simulink model "IEEE14_case"  (R2024b)
settings: Solver=FixedStepAuto  StartTime=0  StopTime=2  FixedStep=1e-7  RelTol=1e-3
values from neighbouring files (symbols this model uses):
  GFL_15_Bva = 0.009    [IEEE14_parameters.m]
  GFL_15_C_bus_pu = 7.179419    [IEEE14_parameters.m]
  GFL_15_f0 = 60    [IEEE14_parameters.m]
  GFL_15_I_id = 691.26967    [IEEE14_parameters.m]
  GFL_15_I_iq = 691.26967    [IEEE14_parameters.m]
  GFL_15_I_od = 45.2207    [IEEE14_parameters.m]
  GFL_15_I_oq = 45.2207    [IEEE14_parameters.m]
  GFL_15_I_pll = 0.78    [IEEE14_parameters.m]
  GFL_15_Kdi = 0.09    [IEEE14_parameters.m]
  GFL_15_Kdo = 0.9    [IEEE14_parameters.m]
  GFL_15_Kqi = 0.09    [IEEE14_parameters.m]
  GFL_15_Kqo = 0.9    [IEEE14_parameters.m]
  GFL_15_Lg_pu = 0.631447    [IEEE14_parameters.m]
  GFL_15_mode = 1    [IEEE14_parameters.m]
  GFL_15_P_id = 3.7166    [IEEE14_parameters.m]
  GFL_15_P_iq = 3.7166    [IEEE14_parameters.m]
  GFL_15_P_od = 0.4798    [IEEE14_parameters.m]
  GFL_15_P_oq = 0.4798    [IEEE14_parameters.m]
  GFL_15_P_pll = 290.42    [IEEE14_parameters.m]
  GFL_15_Qe_ref = 0.2    [IEEE14_parameters.m]
  GFL_15_Rg_pu = 0.024016    [IEEE14_parameters.m]
  GFL_15_Sbase = 1.000000e+4    (= 10000)    [IEEE14_parameters.m]
  GFL_15_Tdi = 0.01    [IEEE14_parameters.m]
  GFL_15_Tdo = 0.2    [IEEE14_parameters.m]
  GFL_15_Tqi = 0.01    [IEEE14_parameters.m]
  GFL_15_Tqo = 0.2    [IEEE14_parameters.m]
  GFL_15_Vbase = 380    [IEEE14_parameters.m]
  GFL_15_Vdc_ref = 1.011475    [IEEE14_parameters.m]
  GFL_15_Vdcbase = 700    [IEEE14_parameters.m]
  GFL_15_vq_ref = 0    [IEEE14_parameters.m]
  GFL_16_Bva = 0.002    [IEEE14_parameters.m]
  GFL_16_C_bus_pu = 7.179419    [IEEE14_parameters.m]
  GFL_16_f0 = 60    [IEEE14_parameters.m]
  GFL_16_I_id = 691.26967    [IEEE14_parameters.m]
  GFL_16_I_iq = 691.26967    [IEEE14_parameters.m]
  GFL_16_I_od = 45.2207    [IEEE14_parameters.m]
  GFL_16_I_oq = 45.2207    [IEEE14_parameters.m]
  GFL_16_I_pll = 0.78    [IEEE14_parameters.m]
  GFL_16_Kdi = 0.05    [IEEE14_parameters.m]
  GFL_16_Kdo = 0.5    [IEEE14_parameters.m]
  GFL_16_Kqi = 0.05    [IEEE14_parameters.m]
  GFL_16_Kqo = 0.5    [IEEE14_parameters.m]
  GFL_16_Lg_pu = 0.631447    [IEEE14_parameters.m]
  GFL_16_mode = 1    [IEEE14_parameters.m]
  GFL_16_P_id = 3.7166    [IEEE14_parameters.m]
  GFL_16_P_iq = 3.7166    [IEEE14_parameters.m]
  GFL_16_P_od = 0.4798    [IEEE14_parameters.m]
  GFL_16_P_oq = 0.4798    [IEEE14_parameters.m]
  GFL_16_P_pll = 290.42    [IEEE14_parameters.m]
  GFL_16_Qe_ref = 0.2    [IEEE14_parameters.m]
  GFL_16_Rg_pu = 0.024016    [IEEE14_parameters.m]
  GFL_16_Sbase = 1.000000e+4    (= 10000)    [IEEE14_parameters.m]
  GFL_16_Tdi = 0.01    [IEEE14_parameters.m]
  GFL_16_Tdo = 0.2    [IEEE14_parameters.m]
  GFL_16_Tqi = 0.01    [IEEE14_parameters.m]
  GFL_16_Tqo = 0.2    [IEEE14_parameters.m]
  GFL_16_Vbase = 380    [IEEE14_parameters.m]
  GFL_16_Vdc_ref = 1.01144    [IEEE14_parameters.m]
  GFL_16_Vdcbase = 700    [IEEE14_parameters.m]
  GFL_16_vq_ref = 0    [IEEE14_parameters.m]
  GFL_17_Bva = 0.002    [IEEE14_parameters.m]
  GFL_17_C_bus_pu = 7.179419    [IEEE14_parameters.m]
  GFL_17_f0 = 60    [IEEE14_parameters.m]
  GFL_17_I_id = 691.26967    [IEEE14_parameters.m]
  GFL_17_I_iq = 691.26967    [IEEE14_parameters.m]
  GFL_17_I_od = 45.2207    [IEEE14_parameters.m]
  GFL_17_I_oq = 45.2207    [IEEE14_parameters.m]
  GFL_17_I_pll = 0.78    [IEEE14_parameters.m]
  GFL_17_Kdi = 0.05    [IEEE14_parameters.m]
  GFL_17_Kdo = 0.5    [IEEE14_parameters.m]
  GFL_17_Kqi = 0.05    [IEEE14_parameters.m]
  GFL_17_Kqo = 0.5    [IEEE14_parameters.m]
  GFL_17_Lg_pu = 0.631447    [IEEE14_parameters.m]
  GFL_17_mode = 1    [IEEE14_parameters.m]
  GFL_17_P_id = 3.7166    [IEEE14_parameters.m]
  GFL_17_P_iq = 3.7166    [IEEE14_parameters.m]
  GFL_17_P_od = 0.4798    [IEEE14_parameters.m]
  GFL_17_P_oq = 0.4798    [IEEE14_parameters.m]
  GFL_17_P_pll = 290.42    [IEEE14_parameters.m]
  GFL_17_Qe_ref = 0.2    [IEEE14_parameters.m]
  GFL_17_Rg_pu = 0.024016    [IEEE14_parameters.m]
  GFL_17_Sbase = 1.000000e+4    (= 10000)    [IEEE14_parameters.m]
  GFL_17_Tdi = 0.01    [IEEE14_parameters.m]
  GFL_17_Tdo = 0.2    [IEEE14_parameters.m]
  GFL_17_Tqi = 0.01    [IEEE14_parameters.m]
  GFL_17_Tqo = 0.2    [IEEE14_parameters.m]
  GFL_17_Vbase = 380    [IEEE14_parameters.m]
  GFL_17_Vdc_ref = 1.011632    [IEEE14_parameters.m]
  GFL_17_Vdcbase = 700    [IEEE14_parameters.m]
  GFL_17_vq_ref = 0    [IEEE14_parameters.m]
  GFL_18_Bva = 0.002    [IEEE14_parameters.m]
  GFL_18_C_bus_pu = 7.179419    [IEEE14_parameters.m]
  GFL_18_f0 = 60    [IEEE14_parameters.m]
  GFL_18_I_id = 691.26967    [IEEE14_parameters.m]
  GFL_18_I_iq = 691.26967    [IEEE14_parameters.m]
  GFL_18_I_od = 45.2207    [IEEE14_parameters.m]
  GFL_18_I_oq = 45.2207    [IEEE14_parameters.m]
  GFL_18_I_pll = 0.78    [IEEE14_parameters.m]
  GFL_18_Kdi = 0.05    [IEEE14_parameters.m]
  GFL_18_Kdo = 0.5    [IEEE14_parameters.m]
  GFL_18_Kqi = 0.05    [IEEE14_parameters.m]
  GFL_18_Kqo = 0.5    [IEEE14_parameters.m]
  GFL_18_Lg_pu = 0.631447    [IEEE14_parameters.m]
  GFL_18_mode = 1    [IEEE14_parameters.m]
  GFL_18_P_id = 3.7166    [IEEE14_parameters.m]
  GFL_18_P_iq = 3.7166    [IEEE14_parameters.m]
  GFL_18_P_od = 0.4798    [IEEE14_parameters.m]
  GFL_18_P_oq = 0.4798    [IEEE14_parameters.m]
  GFL_18_P_pll = 290.42    [IEEE14_parameters.m]
  GFL_18_Qe_ref = 0.2    [IEEE14_parameters.m]
  GFL_18_Rg_pu = 0.024016    [IEEE14_parameters.m]
  GFL_18_Sbase = 1.000000e+4    (= 10000)    [IEEE14_parameters.m]
  GFL_18_Tdi = 0.01    [IEEE14_parameters.m]
  GFL_18_Tdo = 0.2    [IEEE14_parameters.m]
  GFL_18_Tqi = 0.01    [IEEE14_parameters.m]
  GFL_18_Tqo = 0.2    [IEEE14_parameters.m]
  GFL_18_Vbase = 380    [IEEE14_parameters.m]
  GFL_18_Vdc_ref = 1.011572    [IEEE14_parameters.m]
  GFL_18_Vdcbase = 700    [IEEE14_parameters.m]
  GFL_18_vq_ref = 0    [IEEE14_parameters.m]
  ... (+180 more)
(part 9 of 25)

== system IEEE14_case/AC_1/iq_bus_6_block ==
  note: iq_bus_6 in case14gfl
      | $\mathrm{iq}_{\mathrm{SG},D,6}-\mathrm{iq}_{\mathrm{load},6}+\mathrm{iq}_{\mathrm{line},5,6}-\mathrm{iq}_{\mathrm{line},6,11}-\mathrm{iq}_{\mathrm{line},6,12}-\mathrm{iq}_{\mathrm{line},6,13}$
      | Automatically generated on 2025-10-09 21:40:16 .
  Input_iq_SG_D_6_fd9b5 : Inport
  State_iq_load_6_74227 : Inport  Port=2
  State_iq_line_5_6_4236b : Inport  Port=3
  State_iq_line_6_11_dc417 : Inport  Port=4
  State_iq_line_6_12_b02a7 : Inport  Port=5
  State_iq_line_6_13_efd13 : Inport  Port=6
  Add_7536a : Sum
  Subtract_448e5 : Sum  Inputs=+-
  Subtract_74d5f : Sum  Inputs=+-
  Subtract_a35fe : Sum  Inputs=+-
  Subtract_b4e0a : Sum  Inputs=+-
  Blockout_iq_bus_6_4d630 : Outport
  wires:
  Subtract_74d5f/1 -> Subtract_b4e0a/1
  Subtract_a35fe/1 -> Subtract_74d5f/1
  Input_iq_SG_D_6_fd9b5/1 -> Subtract_448e5/1
  Subtract_448e5/1 -> Add_7536a/1
  Add_7536a/1 -> Subtract_a35fe/1
  State_iq_line_5_6_4236b/1 -> Add_7536a/2
  State_iq_load_6_74227/1 -> Subtract_448e5/2
  State_iq_line_6_11_dc417/1 -> Subtract_a35fe/2
  State_iq_line_6_12_b02a7/1 -> Subtract_74d5f/2
  State_iq_line_6_13_efd13/1 -> Subtract_b4e0a/2
  Subtract_b4e0a/1 -> Blockout_iq_bus_6_4d630/1

== system IEEE14_case/AC_1/iq_bus_7_block ==
  note: iq_bus_7 in case14gfl
      | $\mathrm{iq}_{\mathrm{line},4,7}-\mathrm{iq}_{\mathrm{line},7,8}-\mathrm{iq}_{\mathrm{line},7,9}$
      | Automatically generated on 2025-10-09 21:40:18 .
  State_iq_line_4_7_bfb83 : Inport
  State_iq_line_7_8_54428 : Inport  Port=2
  State_iq_line_7_9_fd2c4 : Inport  Port=3
  Subtract_8d108 : Sum  Inputs=+-
  Subtract_ae24a : Sum  Inputs=+-
  Blockout_iq_bus_7_85d72 : Outport
  wires:
  Subtract_8d108/1 -> Blockout_iq_bus_7_85d72/1
  State_iq_line_7_9_fd2c4/1 -> Subtract_8d108/2
  State_iq_line_4_7_bfb83/1 -> Subtract_ae24a/1
  State_iq_line_7_8_54428/1 -> Subtract_ae24a/2
  Subtract_ae24a/1 -> Subtract_8d108/1

== system IEEE14_case/AC_1/iq_bus_8_block ==
  note: iq_bus_8 in case14gfl
      | $\mathrm{iq}_{\mathrm{SG},D,8}+\mathrm{iq}_{\mathrm{line},7,8}$
      | Automatically generated on 2025-10-09 21:40:20 .
  Input_iq_SG_D_8_05cc5 : Inport
  State_iq_line_7_8_02a2e : Inport  Port=2
  Add_2cb00 : Sum
  Blockout_iq_bus_8_a9e89 : Outport
  wires:
  Add_2cb00/1 -> Blockout_iq_bus_8_a9e89/1
  State_iq_line_7_8_02a2e/1 -> Add_2cb00/2
  Input_iq_SG_D_8_05cc5/1 -> Add_2cb00/1

== system IEEE14_case/AC_1/iq_bus_9_block ==
  note: iq_bus_9 in case14gfl
      | $\mathrm{iq}_{\mathrm{line},4,9}-\mathrm{iq}_{\mathrm{load},9}+\mathrm{iq}_{\mathrm{line},7,9}-\mathrm{iq}_{\mathrm{line},9,10}-\mathrm{iq}_{\mathrm{line},9,14}$
      | Automatically generated on 2025-10-09 21:40:22 .
  State_iq_load_9_b0a53 : Inport
  State_iq_line_4_9_4d417 : Inport  Port=2
  State_iq_line_7_9_360e6 : Inport  Port=3
  State_iq_line_9_10_294ee : Inport  Port=4
  State_iq_line_9_14_10f53 : Inport  Port=5
  Add_23a6a : Sum
  Add_e8f35 : Sum
  Constant_-1_d914d : Constant  Value=-1
  Product_e44f7 : Product
  Subtract_3c9e7 : Sum  Inputs=+-
  Subtract_96d13 : Sum  Inputs=+-
  Blockout_iq_bus_9_d3dd5 : Outport
  wires:
  Constant_-1_d914d/1 -> Product_e44f7/1
  Product_e44f7/1 -> Add_23a6a/1
  Add_23a6a/1 -> Add_e8f35/1
  State_iq_line_4_9_4d417/1 -> Add_23a6a/2
  State_iq_load_9_b0a53/1 -> Product_e44f7/2
  State_iq_line_7_9_360e6/1 -> Add_e8f35/2
  Add_e8f35/1 -> Subtract_96d13/1
  State_iq_line_9_10_294ee/1 -> Subtract_96d13/2
  Subtract_96d13/1 -> Subtract_3c9e7/1
  State_iq_line_9_14_10f53/1 -> Subtract_3c9e7/2
  Subtract_3c9e7/1 -> Blockout_iq_bus_9_d3dd5/1

== system IEEE14_case/AC_1/vd_bus_15_out_block ==
  note: vd_bus_15_out in case14gfl
      | $\mathrm{vd}_{\mathrm{bus},15}$
      | Automatically generated on 2025-10-09 21:40:32 .
  State_vd_bus_15_8a646 : Inport
  Blockout_vd_bus_15_out_53236 : Outport
  wires:
  State_vd_bus_15_8a646/1 -> Blockout_vd_bus_15_out_53236/1

== system IEEE14_case/AC_1/vd_bus_16_out_block ==
  note: vd_bus_16_out in case14gfl
      | $\mathrm{vd}_{\mathrm{bus},16}$
      | Automatically generated on 2025-10-09 21:40:34 .
  State_vd_bus_16_c68f5 : Inport
  Blockout_vd_bus_16_out_bf920 : Outport
  wires:
  State_vd_bus_16_c68f5/1 -> Blockout_vd_bus_16_out_bf920/1

== system IEEE14_case/AC_1/vd_bus_17_out_block ==
  note: vd_bus_17_out in case14gfl
      | $\mathrm{vd}_{\mathrm{bus},17}$
      | Automatically generated on 2025-10-09 21:40:37 .
  State_vd_bus_17_d959d : Inport
  Blockout_vd_bus_17_out_ee528 : Outport
  wires:
  State_vd_bus_17_d959d/1 -> Blockout_vd_bus_17_out_ee528/1

== system IEEE14_case/AC_1/vd_bus_18_out_block ==
  note: vd_bus_18_out in case14gfl
      | $\mathrm{vd}_{\mathrm{bus},18}$
      | Automatically generated on 2025-10-09 21:40:40 .
  State_vd_bus_18_46c9f : Inport
  Blockout_vd_bus_18_out_c2e2f : Outport
  wires:
  State_vd_bus_18_46c9f/1 -> Blockout_vd_bus_18_out_c2e2f/1

== system IEEE14_case/AC_1/vd_bus_1_out_block ==
  note: vd_bus_1_out in case14gfl
      | $\mathrm{vd}_{\mathrm{bus},1}$
      | Automatically generated on 2025-10-09 21:40:02 .
  State_vd_bus_1_5dc0e : Inport
  Blockout_vd_bus_1_out_41eef : Outport
  wires:
  State_vd_bus_1_5dc0e/1 -> Blockout_vd_bus_1_out_41eef/1

== system IEEE14_case/AC_1/vd_bus_2_out_block ==
  note: vd_bus_2_out in case14gfl
      | $\mathrm{vd}_{\mathrm{bus},2}$
      | Automatically generated on 2025-10-09 21:40:04 .
  State_vd_bus_2_3f94d : Inport
  Blockout_vd_bus_2_out_d1efc : Outport
  wires:
  State_vd_bus_2_3f94d/1 -> Blockout_vd_bus_2_out_d1efc/1

== system IEEE14_case/AC_1/vd_bus_3_out_block ==
  note: vd_bus_3_out in case14gfl
      | $\mathrm{vd}_{\mathrm{bus},3}$
      | Automatically generated on 2025-10-09 21:40:07 .
  State_vd_bus_3_4d21d : Inport
  Blockout_vd_bus_3_out_e3de8 : Outport
  wires:
  State_vd_bus_3_4d21d/1 -> Blockout_vd_bus_3_out_e3de8/1

== system IEEE14_case/AC_1/vd_bus_6_out_block ==
  note: vd_bus_6_out in case14gfl
      | $\mathrm{vd}_{\mathrm{bus},6}$
      | Automatically generated on 2025-10-09 21:40:14 .
  State_vd_bus_6_a4f60 : Inport
  Blockout_vd_bus_6_out_fb39e : Outport
  wires:
  State_vd_bus_6_a4f60/1 -> Blockout_vd_bus_6_out_fb39e/1

== system IEEE14_case/AC_1/vd_bus_8_out_block ==
  note: vd_bus_8_out in case14gfl
      | $\mathrm{vd}_{\mathrm{bus},8}$
      | Automatically generated on 2025-10-09 21:40:18 .
  State_vd_bus_8_bc007 : Inport
  Blockout_vd_bus_8_out_d3476 : Outport
  wires:
  State_vd_bus_8_bc007/1 -> Blockout_vd_bus_8_out_d3476/1

== system IEEE14_case/AC_1/vq_bus_15_out_block ==
  note: vq_bus_15_out in case14gfl
      | $\mathrm{vq}_{\mathrm{bus},15}$
      | Automatically generated on 2025-10-09 21:40:32 .
  State_vq_bus_15_e85b0 : Inport
  Blockout_vq_bus_15_out_b5487 : Outport
  wires:
  State_vq_bus_15_e85b0/1 -> Blockout_vq_bus_15_out_b5487/1

== system IEEE14_case/AC_1/vq_bus_16_out_block ==
  note: vq_bus_16_out in case14gfl
      | $\mathrm{vq}_{\mathrm{bus},16}$
      | Automatically generated on 2025-10-09 21:40:35 .
  State_vq_bus_16_bbd15 : Inport
  Blockout_vq_bus_16_out_7f446 : Outport
  wires:
  State_vq_bus_16_bbd15/1 -> Blockout_vq_bus_16_out_7f446/1

== system IEEE14_case/AC_1/vq_bus_17_out_block ==
  note: vq_bus_17_out in case14gfl
      | $\mathrm{vq}_{\mathrm{bus},17}$
      | Automatically generated on 2025-10-09 21:40:37 .
  State_vq_bus_17_ceb31 : Inport
  Blockout_vq_bus_17_out_c5b42 : Outport
  wires:
  State_vq_bus_17_ceb31/1 -> Blockout_vq_bus_17_out_c5b42/1

== system IEEE14_case/AC_1/vq_bus_18_out_block ==
  note: vq_bus_18_out in case14gfl
      | $\mathrm{vq}_{\mathrm{bus},18}$
      | Automatically generated on 2025-10-09 21:40:40 .
  State_vq_bus_18_e31db : Inport
  Blockout_vq_bus_18_out_45376 : Outport
  wires:
  State_vq_bus_18_e31db/1 -> Blockout_vq_bus_18_out_45376/1

== system IEEE14_case/AC_1/vq_bus_1_out_block ==
  note: vq_bus_1_out in case14gfl
      | $\mathrm{vq}_{\mathrm{bus},1}$
      | Automatically generated on 2025-10-09 21:40:03 .
  State_vq_bus_1_00178 : Inport
  Blockout_vq_bus_1_out_08423 : Outport
  wires:
  State_vq_bus_1_00178/1 -> Blockout_vq_bus_1_out_08423/1

== system IEEE14_case/AC_1/vq_bus_2_out_block ==
  note: vq_bus_2_out in case14gfl
      | $\mathrm{vq}_{\mathrm{bus},2}$
      | Automatically generated on 2025-10-09 21:40:05 .
  State_vq_bus_2_ea0d1 : Inport
  Blockout_vq_bus_2_out_c2eb9 : Outport
  wires:
  State_vq_bus_2_ea0d1/1 -> Blockout_vq_bus_2_out_c2eb9/1

== system IEEE14_case/AC_1/vq_bus_3_out_block ==
  note: vq_bus_3_out in case14gfl
      | $\mathrm{vq}_{\mathrm{bus},3}$
      | Automatically generated on 2025-10-09 21:40:08 .
  State_vq_bus_3_c1e3e : Inport
  Blockout_vq_bus_3_out_bf333 : Outport
  wires:
  State_vq_bus_3_c1e3e/1 -> Blockout_vq_bus_3_out_bf333/1

== system IEEE14_case/AC_1/vq_bus_6_out_block ==
  note: vq_bus_6_out in case14gfl
      | $\mathrm{vq}_{\mathrm{bus},6}$
      | Automatically generated on 2025-10-09 21:40:14 .
  State_vq_bus_6_b99ed : Inport
  Blockout_vq_bus_6_out_b9abb : Outport
  wires:
  State_vq_bus_6_b99ed/1 -> Blockout_vq_bus_6_out_b9abb/1

== system IEEE14_case/AC_1/vq_bus_8_out_block ==
  note: vq_bus_8_out in case14gfl
      | $\mathrm{vq}_{\mathrm{bus},8}$
      | Automatically generated on 2025-10-09 21:40:19 .
  State_vq_bus_8_b3a86 : Inport
  Blockout_vq_bus_8_out_36371 : Outport
  wires:
  State_vq_bus_8_b3a86/1 -> Blockout_vq_bus_8_out_36371/1

== system IEEE14_case/GFL_15/d_Idv_GFL_15_block ==
  note: d_Idv_GFL_15 in case14gfl
      | $-\frac{\mathrm{Idv}_{\mathrm{GFL},15}+\mathrm{Kdo}\,\left(\mathrm{Vbase}\,\left(v_{q,\mathrm{GFL},15}\,\cos\left(\theta _{\mathrm{pll},\mathrm{GFL},15}\right)+v_{d,\mathrm{GFL},15}\,\sin\left(\theta _{\mathrm{pll},\mathrm{GFL},15}\right)\right)+\frac{\Psi _{d,\mathrm{GFL},15}+\mathrm{Kdi}\,\mathrm{Vbase}\,\left(v_{q,\mathrm{GFL},15}\,\cos\left(\theta _{\mathrm{pll},\mathrm{GFL},15}\right)+v_{d,\mathrm{GFL},15}\,\sin\left(\theta _{\mathrm{pll},\mathrm{GFL},15}\right)\right)}{\mathrm{Tdi}}\right)}{\mathrm{Tdo}}$
      | Automatically generated on 2025-10-09 21:35:26 .
  State_Idv_GFL_15_ca6d1 : Inport
  Input_v_d_GFL_15_d6ef0 : Inport  Port=2
  State_theta_pll_GFL_15_12ffd : Inport  Port=3
  Input_v_q_GFL_15_617c4 : Inport  Port=4
  State_theta_pll_GFL_15_9725f : Inport  Port=5
  Input_v_d_GFL_15_adaa4 : Inport  Port=6
  State_theta_pll_GFL_15_963fe : Inport  Port=7
  Input_v_q_GFL_15_86e6c : Inport  Port=8
  State_theta_pll_GFL_15_2202b : Inport  Port=9
  State_Psi_d_GFL_15_22a12 : Inport  Port=10
  Add_30c23 : Sum
  Add_6e6b0 : Sum
  Add_ecf0e : Sum
  Add_ed6d2 : Sum
  Constant_-1_8c527 : Constant  Value=-1
  Constant_-1_bad54 : Constant  Value=-1
  Constant_-1_d2cc2 : Constant  Value=-1
  Constant_Kdi_3c48e : Constant  Value=Kdi
  Constant_Kdo_c5a85 : Constant  Value=Kdo
  Constant_Tdi_93e84 : Constant  Value=Tdi
  Constant_Tdo_322af : Constant  Value=Tdo
  Constant_Vbase_69f49 : Constant  Value=Vbase
  Constant_Vbase_8e2e0 : Constant  Value=Vbase
  Divide_08330 : Product  Inputs=*/
  Divide_106bd : Product  Inputs=*/
  MathFunc_cos_6a27c : Trigonometry  Operator=cos
  MathFunc_cos_b8fe7 : Trigonometry  Operator=cos
  MathFunc_sin_2b1dd : Trigonometry
  MathFunc_sin_32677 : Trigonometry
  Product_134c0 : Product
  Product_1d184 : Product
  Product_32e14 : Product
  Product_6e7d5 : Product
  Product_75262 : Product
  Product_a160a : Product
  Product_ae5a0 : Product
  Product_beb8a : Product
  Product_d484f : Product
  Product_e74b0 : Product
  Product_f9eeb : Product
  Subtract_37e01 : Sum  Inputs=+-
  Blockout_d_Idv_GFL_15_06d8e : Outport
  wires:
  Add_30c23/1 -> Divide_106bd/1
  State_theta_pll_GFL_15_963fe/1 -> MathFunc_sin_2b1dd/1
  MathFunc_sin_2b1dd/1 -> Product_ae5a0/2
  State_theta_pll_GFL_15_2202b/1 -> MathFunc_cos_6a27c/1
  MathFunc_cos_6a27c/1 -> Product_a160a/2
  Product_1d184/1 -> Add_ed6d2/1
  Constant_Kdi_3c48e/1 -> Product_134c0/2
  Constant_-1_bad54/1 -> Product_134c0/1
  Product_ae5a0/1 -> Add_ecf0e/1
  Input_v_d_GFL_15_adaa4/1 -> Product_ae5a0/1
  Input_v_q_GFL_15_86e6c/1 -> Product_a160a/1
  MathFunc_sin_32677/1 -> Product_1d184/2
  State_theta_pll_GFL_15_12ffd/1 -> MathFunc_sin_32677/1
  State_theta_pll_GFL_15_9725f/1 -> MathFunc_cos_b8fe7/1
  State_Idv_GFL_15_ca6d1/1 -> Product_e74b0/2
  Product_134c0/1 -> Product_32e14/1
  Input_v_d_GFL_15_d6ef0/1 -> Product_1d184/1
  Constant_Vbase_8e2e0/1 -> Product_32e14/2
  Product_a160a/1 -> Add_ecf0e/2
  Input_v_q_GFL_15_617c4/1 -> Product_beb8a/1
  MathFunc_cos_b8fe7/1 -> Product_beb8a/2
  Product_32e14/1 -> Product_d484f/1
  Add_ecf0e/1 -> Product_d484f/2
  Constant_-1_d2cc2/1 -> Product_f9eeb/1
  Constant_Vbase_69f49/1 -> Product_f9eeb/2
  Product_beb8a/1 -> Add_ed6d2/2
  Product_d484f/1 -> Subtract_37e01/1
  State_Psi_d_GFL_15_22a12/1 -> Subtract_37e01/2
  Product_f9eeb/1 -> Product_6e7d5/1
  Add_ed6d2/1 -> Product_6e7d5/2
  Subtract_37e01/1 -> Divide_08330/1
  Constant_Tdi_93e84/1 -> Divide_08330/2
  Product_6e7d5/1 -> Add_6e6b0/1
  Divide_08330/1 -> Add_6e6b0/2
  Constant_-1_8c527/1 -> Product_e74b0/1
  Product_75262/1 -> Add_30c23/2
  Constant_Kdo_c5a85/1 -> Product_75262/1
  Add_6e6b0/1 -> Product_75262/2
  Product_e74b0/1 -> Add_30c23/1
  Constant_Tdo_322af/1 -> Divide_106bd/2
  Divide_106bd/1 -> Blockout_d_Idv_GFL_15_06d8e/1

== system IEEE14_case/GFL_15/d_Iqv_GFL_15_block ==
  note: d_Iqv_GFL_15 in case14gfl
      | $-\frac{\mathrm{Iqv}_{\mathrm{GFL},15}-\mathrm{Kqo}\,\left(\mathrm{Vbase}\,\left(v_{d,\mathrm{GFL},15}\,\cos\left(\theta _{\mathrm{pll},\mathrm{GFL},15}\right)-v_{q,\mathrm{GFL},15}\,\sin\left(\theta _{\mathrm{pll},\mathrm{GFL},15}\right)\right)-\frac{\Psi _{q,\mathrm{GFL},15}-\mathrm{Kqi}\,\mathrm{Vbase}\,\left(v_{d,\mathrm{GFL},15}\,\cos\left(\theta _{\mathrm{pll},\mathrm{GFL},15}\right)-v_{q,\mathrm{GFL},15}\,\sin\left(\theta _{\mathrm{pll},\mathrm{GFL},15}\right)\right)}{\mathrm{Tqi}}\right)}{\mathrm{Tqo}}$
      | Automatically generated on 2025-10-09 21:35:28 .
  State_Iqv_GFL_15_a0efa : Inport
  Input_v_d_GFL_15_e9447 : Inport  Port=2
  State_theta_pll_GFL_15_5bce6 : Inport  Port=3
  Input_v_q_GFL_15_4a34b : Inport  Port=4
  State_theta_pll_GFL_15_c6881 : Inport  Port=5
  Input_v_d_GFL_15_7c93a : Inport  Port=6
  State_theta_pll_GFL_15_e8e0d : Inport  Port=7
  Input_v_q_GFL_15_924af : Inport  Port=8
  State_theta_pll_GFL_15_f624d : Inport  Port=9
  State_Psi_q_GFL_15_d75c1 : Inport  Port=10
  Add_7b66c : Sum
  Add_cf612 : Sum
  Constant_-1_c7459 : Constant  Value=-1
  Constant_Kqi_42f9e : Constant  Value=Kqi
  Constant_Kqo_97ec0 : Constant  Value=Kqo
  Constant_Tqi_2e3dc : Constant  Value=Tqi
  Constant_Tqo_731e7 : Constant  Value=Tqo
  Constant_Vbase_41c60 : Constant  Value=Vbase
  Constant_Vbase_700be : Constant  Value=Vbase
  Divide_61f05 : Product  Inputs=*/
  Divide_b950e : Product  Inputs=*/
  MathFunc_cos_3c92d : Trigonometry  Operator=cos
  MathFunc_cos_c5429 : Trigonometry  Operator=cos
  MathFunc_sin_3ae11 : Trigonometry
  MathFunc_sin_e36a9 : Trigonometry
  Product_13c48 : Product
  Product_2727d : Product
  Product_2c1de : Product
  Product_3cbec : Product
  Product_5de87 : Product
  Product_6c92d : Product
  Product_9c883 : Product
  Product_b238b : Product
  Product_e1ab8 : Product
  Subtract_15861 : Sum  Inputs=+-
  Subtract_84f7c : Sum  Inputs=+-
  Subtract_94af4 : Sum  Inputs=+-
  Blockout_d_Iqv_GFL_15_65918 : Outport
  wires:
  MathFunc_cos_c5429/1 -> Product_5de87/2
  State_theta_pll_GFL_15_5bce6/1 -> MathFunc_cos_c5429/1
  State_theta_pll_GFL_15_e8e0d/1 -> MathFunc_cos_3c92d/1
  MathFunc_sin_3ae11/1 -> Product_b238b/2
  State_theta_pll_GFL_15_c6881/1 -> MathFunc_sin_3ae11/1
  Product_13c48/1 -> Add_7b66c/2
  State_theta_pll_GFL_15_f624d/1 -> MathFunc_sin_e36a9/1
  MathFunc_sin_e36a9/1 -> Product_3cbec/2
  Product_6c92d/1 -> Subtract_15861/1
  Input_v_d_GFL_15_7c93a/1 -> Product_6c92d/1
  MathFunc_cos_3c92d/1 -> Product_6c92d/2
  Product_3cbec/1 -> Subtract_15861/2
  Input_v_q_GFL_15_924af/1 -> Product_3cbec/1
  Product_2727d/1 -> Product_e1ab8/1
  Constant_Kqi_42f9e/1 -> Product_2727d/1
  Constant_Vbase_700be/1 -> Product_2727d/2
  Product_5de87/1 -> Subtract_84f7c/1
  Input_v_d_GFL_15_e9447/1 -> Product_5de87/1
  Input_v_q_GFL_15_4a34b/1 -> Product_b238b/1
  Subtract_15861/1 -> Product_e1ab8/2
  Product_b238b/1 -> Subtract_84f7c/2
  Product_e1ab8/1 -> Subtract_94af4/1
  State_Psi_q_GFL_15_d75c1/1 -> Subtract_94af4/2
  Constant_Vbase_41c60/1 -> Product_9c883/1
  Subtract_84f7c/1 -> Product_9c883/2
  Subtract_94af4/1 -> Divide_b950e/1
  Constant_Tqi_2e3dc/1 -> Divide_b950e/2
  Product_9c883/1 -> Add_cf612/1
  Divide_b950e/1 -> Add_cf612/2
  Constant_-1_c7459/1 -> Product_2c1de/1
  State_Iqv_GFL_15_a0efa/1 -> Product_2c1de/2
  Constant_Kqo_97ec0/1 -> Product_13c48/1
  Add_cf612/1 -> Product_13c48/2
  Divide_61f05/1 -> Blockout_d_Iqv_GFL_15_65918/1
  Product_2c1de/1 -> Add_7b66c/1
  Add_7b66c/1 -> Divide_61f05/1
  Constant_Tqo_731e7/1 -> Divide_61f05/2

== system IEEE14_case/GFL_15/d_Phi_ga_GFL_15_block ==
  note: d_Phi_ga_GFL_15 in case14gfl
      | $I_{\mathrm{od}}\,\left(V_{\mathrm{dc},\mathrm{GFL},15}-\mathrm{Vdcbase}\,\mathrm{Vdc}_{\mathrm{ref}}\right)$
      | Automatically generated on 2025-10-09 21:35:14 .
  State_V_dc_GFL_15_371a8 : Inport
  Constant_I_od_53ece : Constant  Value=I_od
  Constant_Vdc_ref_e5ef2 : Constant  Value=Vdc_ref
  Constant_Vdcbase_c0f83 : Constant  Value=Vdcbase
  Product_b2d23 : Product
  Product_c5cd1 : Product
  Subtract_28544 : Sum  Inputs=+-
  Blockout_d_Phi_ga_GFL_15_ed294 : Outport
  wires:
  Product_c5cd1/1 -> Blockout_d_Phi_ga_GFL_15_ed294/1
  Product_b2d23/1 -> Subtract_28544/2
  Constant_Vdc_ref_e5ef2/1 -> Product_b2d23/1
  Constant_Vdcbase_c0f83/1 -> Product_b2d23/2
  Constant_I_od_53ece/1 -> Product_c5cd1/1
  State_V_dc_GFL_15_371a8/1 -> Subtract_28544/1
  Subtract_28544/1 -> Product_c5cd1/2

== system IEEE14_case/GFL_15/d_Phi_gb_GFL_15_block ==
  note: d_Phi_gb_GFL_15 in case14gfl
      | $I_{\mathrm{id}}\,\left(\mathrm{Idv}_{\mathrm{GFL},15}+\Phi _{\mathrm{ga},\mathrm{GFL},15}-i_{\mathrm{gd},\mathrm{GFL},15}+P_{\mathrm{od}}\,\left(V_{\mathrm{dc},\mathrm{GFL},15}-\mathrm{Vdcbase}\,\mathrm{Vdc}_{\mathrm{ref}}\right)-\mathrm{Bva}\,\mathrm{Vbase}\,\left(v_{d,\mathrm{GFL},15}\,\cos\left(\theta _{\mathrm{pll},\mathrm{GFL},15}\right)-v_{q,\mathrm{GFL},15}\,\sin\left(\theta _{\mathrm{pll},\mathrm{GFL},15}\right)\right)\right)$
      | Automatically generated on 2025-10-09 21:35:15 .
  Input_v_d_GFL_15_ba16a : Inport
  State_theta_pll_GFL_15_82324 : Inport  Port=2
  Input_v_q_GFL_15_e2248 : Inport  Port=3
  State_theta_pll_GFL_15_58522 : Inport  Port=4
  State_Idv_GFL_15_4c70c : Inport  Port=5
  State_V_dc_GFL_15_cf545 : Inport  Port=6
  State_Phi_ga_GFL_15_778c9 : Inport  Port=7
  State_i_gd_GFL_15_ca8ed : Inport  Port=8
  Add_7f088 : Sum
  Add_ba3ac : Sum
  Add_cab57 : Sum
  Constant_-1_d2a66 : Constant  Value=-1
  Constant_Bva_25216 : Constant  Value=Bva
  Constant_I_id_90b40 : Constant  Value=I_id
  Constant_P_od_b2591 : Constant  Value=P_od
  Constant_Vbase_4f081 : Constant  Value=Vbase
  Constant_Vdc_ref_8d8d4 : Constant  Value=Vdc_ref
  Constant_Vdcbase_e266d : Constant  Value=Vdcbase
  MathFunc_cos_073c5 : Trigonometry  Operator=cos
  MathFunc_sin_6f8a0 : Trigonometry
  Product_24fb4 : Product
  Product_2f798 : Product
  Product_574fd : Product
  Product_5845e : Product
  Product_75092 : Product
  Product_77499 : Product
  Product_b1701 : Product
  Product_c7754 : Product
  Subtract_311fa : Sum  Inputs=+-
  Subtract_429b0 : Sum  Inputs=+-
  Subtract_9a423 : Sum  Inputs=+-
  Blockout_d_Phi_gb_GFL_15_f24ee : Outport
  wires:
  MathFunc_cos_073c5/1 -> Product_c7754/2
  State_theta_pll_GFL_15_82324/1 -> MathFunc_cos_073c5/1
  State_theta_pll_GFL_15_58522/1 -> MathFunc_sin_6f8a0/1
  MathFunc_sin_6f8a0/1 -> Product_24fb4/2
  Product_24fb4/1 -> Subtract_9a423/2
  Input_v_q_GFL_15_e2248/1 -> Product_24fb4/1
  Product_5845e/1 -> Product_75092/1
  Constant_-1_d2a66/1 -> Product_5845e/1
  Constant_Bva_25216/1 -> Product_5845e/2
  State_Phi_ga_GFL_15_778c9/1 -> Add_ba3ac/2
  Product_c7754/1 -> Subtract_9a423/1
  Input_v_d_GFL_15_ba16a/1 -> Product_c7754/1
  Constant_Vbase_4f081/1 -> Product_75092/2
  Product_b1701/1 -> Subtract_429b0/2
  Constant_Vdc_ref_8d8d4/1 -> Product_b1701/1
  Constant_Vdcbase_e266d/1 -> Product_b1701/2
  Product_75092/1 -> Product_77499/1
  Subtract_9a423/1 -> Product_77499/2
  Subtract_429b0/1 -> Product_2f798/2
  State_V_dc_GFL_15_cf545/1 -> Subtract_429b0/1
  Product_77499/1 -> Add_cab57/1
  State_Idv_GFL_15_4c70c/1 -> Add_cab57/2
  Product_2f798/1 -> Add_7f088/2
  Constant_P_od_b2591/1 -> Product_2f798/1
  Add_cab57/1 -> Add_7f088/1
  Add_7f088/1 -> Add_ba3ac/1
  Add_ba3ac/1 -> Subtract_311fa/1
  State_i_gd_GFL_15_ca8ed/1 -> Subtract_311fa/2
  Constant_I_id_90b40/1 -> Product_574fd/1
  Subtract_311fa/1 -> Product_574fd/2
  Product_574fd/1 -> Blockout_d_Phi_gb_GFL_15_f24ee/1

== system IEEE14_case/GFL_15/d_Phi_gc_GFL_15_block ==
  note: d_Phi_gc_GFL_15 in case14gfl
      | $-I_{\mathrm{oq}}\,\left(\mathrm{Qe}_{\mathrm{ref}}\,\mathrm{Sbase}+1.73205080756888\,\mathrm{Vbase}\,i_{\mathrm{gd},\mathrm{GFL},15}\,\left(v_{q,\mathrm{GFL},15}\,\cos\left(\theta _{\mathrm{pll},\mathrm{GFL},15}\right)+v_{d,\mathrm{GFL},15}\,\sin\left(\theta _{\mathrm{pll},\mathrm{GFL},15}\right)\right)+1.73205080756888\,\mathrm{Vbase}\,i_{\mathrm{gq},\mathrm{GFL},15}\,\left(v_{d,\mathrm{GFL},15}\,\cos\left(\theta _{\mathrm{pll},\mathrm{GFL},15}\right)-v_{q,\mathrm{GFL},15}\,\sin\left(\theta _{\mathrm{pll},\mathrm{GFL},15}\right)\right)\right)$
      | Automatically generated on 2025-10-09 21:35:18 .
  State_i_gd_GFL_15_68d30 : Inport
  Input_v_d_GFL_15_05f07 : Inport  Port=2
  State_theta_pll_GFL_15_5b93f : Inport  Port=3
  Input_v_q_GFL_15_7ae45 : Inport  Port=4
  State_theta_pll_GFL_15_647bc : Inport  Port=5
  State_i_gq_GFL_15_2aff2 : Inport  Port=6
  Input_v_d_GFL_15_b97ec : Inport  Port=7
  State_theta_pll_GFL_15_01aaa : Inport  Port=8
  Input_v_q_GFL_15_e532d : Inport  Port=9
  State_theta_pll_GFL_15_159ad : Inport  Port=10
  Add_22d89 : Sum
  Constant_-1_9fe09 : Constant  Value=-1
  Constant_1.73205080756888_95c30 : Constant  Value=1.73205080756888
  Constant_1.73205080756888_adc02 : Constant  Value=1.73205080756888
  Constant_I_oq_43684 : Constant  Value=I_oq
  Constant_Qe_ref_39675 : Constant  Value=Qe_ref
  Constant_Sbase_ef90e : Constant  Value=Sbase
  Constant_Vbase_165ac : Constant  Value=Vbase
  Constant_Vbase_444de : Constant  Value=Vbase
  MathFunc_cos_21d53 : Trigonometry  Operator=cos
  MathFunc_cos_37d3c : Trigonometry  Operator=cos
  MathFunc_sin_79138 : Trigonometry
  MathFunc_sin_f75ee : Trigonometry
  Product_056a8 : Product
  Product_33f5c : Product
  Product_3aaee : Product
  Product_3ac96 : Product
  Product_3c8ad : Product
  Product_3fb5a : Product
  Product_40490 : Product
  Product_5409f : Product
  Product_56584 : Product
  Product_9fe54 : Product
  Product_b8d19 : Product
  Product_bcdf0 : Product
  Product_cff74 : Product
  Subtract_2bf23 : Sum  Inputs=+-
  Subtract_5939a : Sum  Inputs=+-
  Subtract_a8f65 : Sum  Inputs=+-
  Blockout_d_Phi_gc_GFL_15_8e044 : Outport
  wires:
  State_theta_pll_GFL_15_5b93f/1 -> MathFunc_sin_f75ee/1
  MathFunc_sin_f75ee/1 -> Product_056a8/2
  State_theta_pll_GFL_15_647bc/1 -> MathFunc_cos_21d53/1
  MathFunc_cos_21d53/1 -> Product_40490/2
  Constant_Vbase_165ac/1 -> Product_3aaee/2
  Product_3aaee/1 -> Product_5409f/1
  Constant_1.73205080756888_adc02/1 -> Product_3aaee/1
  Product_056a8/1 -> Add_22d89/1
  Input_v_d_GFL_15_05f07/1 -> Product_056a8/1
  Input_v_q_GFL_15_7ae45/1 -> Product_40490/1
  MathFunc_cos_37d3c/1 -> Product_9fe54/2
  State_theta_pll_GFL_15_01aaa/1 -> MathFunc_cos_37d3c/1
  State_theta_pll_GFL_15_159ad/1 -> MathFunc_sin_79138/1
  Constant_I_oq_43684/1 -> Product_33f5c/1
  Product_3ac96/1 -> Product_3c8ad/1
  Constant_-1_9fe09/1 -> Product_3ac96/1
  Input_v_d_GFL_15_b97ec/1 -> Product_9fe54/1
  Constant_Qe_ref_39675/1 -> Product_3ac96/2
  State_i_gd_GFL_15_68d30/1 -> Product_5409f/2
  Product_40490/1 -> Add_22d89/2
  Constant_1.73205080756888_95c30/1 -> Product_cff74/1
  MathFunc_sin_79138/1 -> Product_bcdf0/2
  Constant_Vbase_444de/1 -> Product_cff74/2
  Input_v_q_GFL_15_e532d/1 -> Product_bcdf0/1
  Constant_Sbase_ef90e/1 -> Product_3c8ad/2
  Product_3c8ad/1 -> Subtract_2bf23/1
  Product_5409f/1 -> Product_56584/1
  Add_22d89/1 -> Product_56584/2
  Product_cff74/1 -> Product_b8d19/1
  State_i_gq_GFL_15_2aff2/1 -> Product_b8d19/2
  Product_9fe54/1 -> Subtract_a8f65/1
  Product_bcdf0/1 -> Subtract_a8f65/2
  Product_56584/1 -> Subtract_2bf23/2
  Product_b8d19/1 -> Product_3fb5a/1
  Subtract_a8f65/1 -> Product_3fb5a/2
  Product_3fb5a/1 -> Subtract_5939a/2
  Subtract_2bf23/1 -> Subtract_5939a/1
  Subtract_5939a/1 -> Product_33f5c/2
  Product_33f5c/1 -> Blockout_d_Phi_gc_GFL_15_8e044/1

== system IEEE14_case/GFL_15/d_Phi_gd_GFL_15_block ==
  note: d_Phi_gd_GFL_15 in case14gfl
      | $I_{\mathrm{iq}}\,\left(\mathrm{Iqv}_{\mathrm{GFL},15}+\Phi _{\mathrm{gc},\mathrm{GFL},15}-i_{\mathrm{gq},\mathrm{GFL},15}-P_{\mathrm{oq}}\,\left(\mathrm{Qe}_{\mathrm{ref}}\,\mathrm{Sbase}+1.73205080756888\,\mathrm{Vbase}\,i_{\mathrm{gd},\mathrm{GFL},15}\,\left(v_{q,\mathrm{GFL},15}\,\cos\left(\theta _{\mathrm{pll},\mathrm{GFL},15}\right)+v_{d,\mathrm{GFL},15}\,\sin\left(\theta _{\mathrm{pll},\mathrm{GFL},15}\right)\right)+1.73205080756888\,\mathrm{Vbase}\,i_{\mathrm{gq},\mathrm{GFL},15}\,\left(v_{d,\mathrm{GFL},15}\,\cos\left(\theta _{\mathrm{pll},\mathrm{GFL},15}\right)-v_{q,\mathrm{GFL},15}\,\sin\left(\theta _{\mathrm{pll},\mathrm{GFL},15}\right)\right)\right)+\mathrm{Bva}\,\mathrm{Vbase}\,\left(v_{q,\mathrm{GFL},15}\,\cos\left(\theta _{\mathrm{pll},\mathrm{GFL},15}\right)+v_{d,\mathrm{GFL},15}\,\sin\left(\theta _{\mathrm{pll},\mathrm{GFL},15}\right)\right)\right)$
      | Automatically generated on 2025-10-09 21:35:21 .
  Input_v_d_GFL_15_e0c96 : Inport
  State_theta_pll_GFL_15_e398b : Inport  Port=2
  Input_v_q_GFL_15_9f181 : Inport  Port=3
  State_theta_pll_GFL_15_d2b83 : Inport  Port=4
  State_Iqv_GFL_15_f6823 : Inport  Port=5
  State_i_gd_GFL_15_7f54c : Inport  Port=6
  Input_v_d_GFL_15_19381 : Inport  Port=7
  State_theta_pll_GFL_15_37f0e : Inport  Port=8
  Input_v_q_GFL_15_fe173 : Inport  Port=9
  State_theta_pll_GFL_15_ae580 : Inport  Port=10
  State_i_gq_GFL_15_08dfd : Inport  Port=11
  Input_v_d_GFL_15_96988 : Inport  Port=12
  State_theta_pll_GFL_15_e05ad : Inport  Port=13
  Input_v_q_GFL_15_7c25a : Inport  Port=14
  State_theta_pll_GFL_15_0e420 : Inport  Port=15
  State_Phi_gc_GFL_15_d40bd : Inport  Port=16
  State_i_gq_GFL_15_39259 : Inport  Port=17
  Add_8654d : Sum
  Add_8ea35 : Sum
  Add_917b3 : Sum
  Add_e396c : Sum
  Add_f04a2 : Sum
  Constant_-1_85dc4 : Constant  Value=-1
  Constant_1.73205080756888_77875 : Constant  Value=1.73205080756888
  Constant_1.73205080756888_88e3e : Constant  Value=1.73205080756888
  Constant_Bva_34f37 : Constant  Value=Bva
  Constant_I_iq_95aed : Constant  Value=I_iq
  Constant_P_oq_faa5b : Constant  Value=P_oq
  Constant_Qe_ref_a118f : Constant  Value=Qe_ref
  Constant_Sbase_1299d : Constant  Value=Sbase
  Constant_Vbase_56f9e : Constant  Value=Vbase
  Constant_Vbase_7611b : Constant  Value=Vbase
  Constant_Vbase_79ed2 : Constant  Value=Vbase
  MathFunc_cos_44114 : Trigonometry  Operator=cos
  MathFunc_cos_4b93c : Trigonometry  Operator=cos
  MathFunc_cos_9e9ad : Trigonometry  Operator=cos
  MathFunc_sin_0f4fd : Trigonometry
  MathFunc_sin_40b8c : Trigonometry
  MathFunc_sin_aae02 : Trigonometry
  Product_0eaed : Product
  Product_0fd4f : Product
  Product_1a17b : Product
  Product_36f4c : Product
  Product_42ecb : Product
  Product_44658 : Product
  Product_6307b : Product
  Product_69431 : Product
  Product_7287d : Product
  Product_8c547 : Product
  Product_aed95 : Product
  Product_af53e : Product
  Product_bced1 : Product
  Product_cca59 : Product
  Product_db3da : Product
  Product_e0003 : Product
  Product_ed453 : Product
  Product_fbb5b : Product
  Subtract_1efaa : Sum  Inputs=+-
  Subtract_8933a : Sum  Inputs=+-
  Subtract_c0214 : Sum  Inputs=+-
  Subtract_d5004 : Sum  Inputs=+-
  Blockout_d_Phi_gd_GFL_15_84e3d : Outport
  wires:
  State_theta_pll_GFL_15_37f0e/1 -> MathFunc_sin_0f4fd/1
  Product_8c547/1 -> Add_917b3/1
  Input_v_d_GFL_15_e0c96/1 -> Product_8c547/1
  Constant_Vbase_7611b/1 -> Product_42ecb/2
  State_theta_pll_GFL_15_ae580/1 -> MathFunc_cos_9e9ad/1
  Constant_Bva_34f37/1 -> Product_69431/1
  Constant_1.73205080756888_77875/1 -> Product_42ecb/1
  Input_v_d_GFL_15_19381/1 -> Product_0eaed/1
  MathFunc_sin_0f4fd/1 -> Product_0eaed/2
  Product_bced1/1 -> Add_8ea35/2
  Input_v_q_GFL_15_fe173/1 -> Product_bced1/1
  MathFunc_cos_9e9ad/1 -> Product_bced1/2
  State_theta_pll_GFL_15_e05ad/1 -> MathFunc_cos_44114/1
  MathFunc_sin_40b8c/1 -> Product_1a17b/2
  Constant_Vbase_79ed2/1 -> Product_7287d/2
  State_theta_pll_GFL_15_0e420/1 -> MathFunc_sin_40b8c/1
  State_theta_pll_GFL_15_e398b/1 -> MathFunc_sin_aae02/1
  MathFunc_cos_4b93c/1 -> Product_0fd4f/2
  Constant_Qe_ref_a118f/1 -> Product_e0003/2
  State_theta_pll_GFL_15_d2b83/1 -> MathFunc_cos_4b93c/1
  Product_e0003/1 -> Product_db3da/1
  Constant_-1_85dc4/1 -> Product_e0003/1
  Product_42ecb/1 -> Product_aed95/1
  State_i_gd_GFL_15_7f54c/1 -> Product_aed95/2
  Product_af53e/1 -> Add_8654d/1
  Product_0eaed/1 -> Add_8ea35/1
  Product_69431/1 -> Product_af53e/1
  Product_7287d/1 -> Product_44658/1
  Constant_1.73205080756888_88e3e/1 -> Product_7287d/1
  Product_fbb5b/1 -> Subtract_1efaa/1
  Input_v_d_GFL_15_96988/1 -> Product_fbb5b/1
  MathFunc_cos_44114/1 -> Product_fbb5b/2
  Product_1a17b/1 -> Subtract_1efaa/2
  Input_v_q_GFL_15_7c25a/1 -> Product_1a17b/1
  MathFunc_sin_aae02/1 -> Product_8c547/2
  Product_0fd4f/1 -> Add_917b3/2
  Input_v_q_GFL_15_9f181/1 -> Product_0fd4f/1
  Constant_Sbase_1299d/1 -> Product_db3da/2
  Product_aed95/1 -> Product_36f4c/1
  Add_8ea35/1 -> Product_36f4c/2
  Add_8654d/1 -> Add_e396c/1
  State_i_gq_GFL_15_08dfd/1 -> Product_44658/2
  Constant_Vbase_56f9e/1 -> Product_69431/2
  Product_db3da/1 -> Subtract_8933a/1
  Product_36f4c/1 -> Subtract_8933a/2
  Product_44658/1 -> Product_ed453/1
  Subtract_c0214/1 -> Product_6307b/2
  Subtract_1efaa/1 -> Product_ed453/2
  Add_917b3/1 -> Product_af53e/2
  Subtract_8933a/1 -> Subtract_d5004/1
  Product_ed453/1 -> Subtract_d5004/2
  State_Iqv_GFL_15_f6823/1 -> Add_8654d/2
  Product_cca59/1 -> Add_e396c/2
  Constant_P_oq_faa5b/1 -> Product_cca59/1
  Subtract_d5004/1 -> Product_cca59/2
  Add_e396c/1 -> Add_f04a2/1
  State_Phi_gc_GFL_15_d40bd/1 -> Add_f04a2/2
  Add_f04a2/1 -> Subtract_c0214/1
  State_i_gq_GFL_15_39259/1 -> Subtract_c0214/2
  Constant_I_iq_95aed/1 -> Product_6307b/1
  Product_6307b/1 -> Blockout_d_Phi_gd_GFL_15_84e3d/1

== system IEEE14_case/GFL_15/d_Phipll_GFL_15_block ==
  note: d_Phipll_GFL_15 in case14gfl
      | $-I_{\mathrm{pll}}\,\left(\mathrm{vq}_{\mathrm{ref}}+v_{q,\mathrm{GFL},15}\,\cos\left(\theta _{\mathrm{pll},\mathrm{GFL},15}\right)+v_{d,\mathrm{GFL},15}\,\sin\left(\theta _{\mathrm{pll},\mathrm{GFL},15}\right)\right)$
      | Automatically generated on 2025-10-09 21:35:11 .
  Input_v_d_GFL_15_62a1f : Inport
  State_theta_pll_GFL_15_65253 : Inport  Port=2
  Input_v_q_GFL_15_2a56a : Inport  Port=3
  State_theta_pll_GFL_15_facf8 : Inport  Port=4
  Constant_-1_edfa3 : Constant  Value=-1
  Constant_I_pll_51a92 : Constant  Value=I_pll
  Constant_vq_ref_85f17 : Constant  Value=vq_ref
  MathFunc_cos_b339b : Trigonometry  Operator=cos
  MathFunc_sin_cbcbe : Trigonometry
  Product_65245 : Product
  Product_6579f : Product
  Product_8985f : Product
  Product_b6efe : Product
  Subtract_02f16 : Sum  Inputs=+-
  Subtract_d6577 : Sum  Inputs=+-
  Blockout_d_Phipll_GFL_15_2e0e5 : Outport
  wires:
  State_theta_pll_GFL_15_facf8/1 -> MathFunc_cos_b339b/1
  Constant_-1_edfa3/1 -> Product_65245/1
  Input_v_d_GFL_15_62a1f/1 -> Product_65245/2
  Subtract_02f16/1 -> Product_8985f/2
  Input_v_q_GFL_15_2a56a/1 -> Product_6579f/1
  Constant_I_pll_51a92/1 -> Product_8985f/1
  State_theta_pll_GFL_15_65253/1 -> MathFunc_sin_cbcbe/1
  MathFunc_sin_cbcbe/1 -> Product_b6efe/2
  Product_65245/1 -> Product_b6efe/1
  MathFunc_cos_b339b/1 -> Product_6579f/2
  Product_b6efe/1 -> Subtract_d6577/1
  Product_6579f/1 -> Subtract_d6577/2
  Subtract_d6577/1 -> Subtract_02f16/1
  Constant_vq_ref_85f17/1 -> Subtract_02f16/2
  Product_8985f/1 -> Blockout_d_Phipll_GFL_15_2e0e5/1

== system IEEE14_case/GFL_15/d_Psi_d_GFL_15_block ==
  note: d_Psi_d_GFL_15 in case14gfl
      | $-\frac{\Psi _{d,\mathrm{GFL},15}+\mathrm{Kdi}\,\mathrm{Vbase}\,\left(v_{q,\mathrm{GFL},15}\,\cos\left(\theta _{\mathrm{pll},\mathrm{GFL},15}\right)+v_{d,\mathrm{GFL},15}\,\sin\left(\theta _{\mathrm{pll},\mathrm{GFL},15}\right)\right)}{\mathrm{Tdi}}$
      | Automatically generated on 2025-10-09 21:35:22 .
  Input_v_d_GFL_15_d26c2 : Inport
  State_theta_pll_GFL_15_95588 : Inport  Port=2
  Input_v_q_GFL_15_84d7e : Inport  Port=3
  State_theta_pll_GFL_15_90724 : Inport  Port=4
  State_Psi_d_GFL_15_90def : Inport  Port=5
  Add_cdf74 : Sum
  Constant_-1_699f6 : Constant  Value=-1
  Constant_Kdi_c5769 : Constant  Value=Kdi
  Constant_Tdi_9170d : Constant  Value=Tdi
  Constant_Vbase_33e89 : Constant  Value=Vbase
  Divide_c13e3 : Product  Inputs=*/
  MathFunc_cos_7d910 : Trigonometry  Operator=cos
  MathFunc_sin_3c6b2 : Trigonometry
  Product_06276 : Product
  Product_0a238 : Product
  Product_6d962 : Product
  Product_91339 : Product
  Product_a035a : Product
  Subtract_78426 : Sum  Inputs=+-
  Blockout_d_Psi_d_GFL_15_bd2bd : Outport
  wires:
  MathFunc_sin_3c6b2/1 -> Product_0a238/2
  Constant_Kdi_c5769/1 -> Product_06276/2
  State_theta_pll_GFL_15_95588/1 -> MathFunc_sin_3c6b2/1
  Input_v_d_GFL_15_d26c2/1 -> Product_0a238/1
  State_theta_pll_GFL_15_90724/1 -> MathFunc_cos_7d910/1
  Input_v_q_GFL_15_84d7e/1 -> Product_a035a/1
  Constant_-1_699f6/1 -> Product_06276/1
  MathFunc_cos_7d910/1 -> Product_a035a/2
  Product_06276/1 -> Product_6d962/1
  Constant_Vbase_33e89/1 -> Product_6d962/2
  Product_0a238/1 -> Add_cdf74/1
  Product_a035a/1 -> Add_cdf74/2
  Product_6d962/1 -> Product_91339/1
  Add_cdf74/1 -> Product_91339/2
  Product_91339/1 -> Subtract_78426/1
  State_Psi_d_GFL_15_90def/1 -> Subtract_78426/2
  Subtract_78426/1 -> Divide_c13e3/1
  Constant_Tdi_9170d/1 -> Divide_c13e3/2
  Divide_c13e3/1 -> Blockout_d_Psi_d_GFL_15_bd2bd/1

== system IEEE14_case/GFL_15/d_Psi_q_GFL_15_block ==
  note: d_Psi_q_GFL_15 in case14gfl
      | $-\frac{\Psi _{q,\mathrm{GFL},15}-\mathrm{Kqi}\,\mathrm{Vbase}\,\left(v_{d,\mathrm{GFL},15}\,\cos\left(\theta _{\mathrm{pll},\mathrm{GFL},15}\right)-v_{q,\mathrm{GFL},15}\,\sin\left(\theta _{\mathrm{pll},\mathrm{GFL},15}\right)\right)}{\mathrm{Tqi}}$
      | Automatically generated on 2025-10-09 21:35:24 .
  Input_v_d_GFL_15_07bda : Inport
  State_theta_pll_GFL_15_42098 : Inport  Port=2
  Input_v_q_GFL_15_da40e : Inport  Port=3
  State_theta_pll_GFL_15_5b172 : Inport  Port=4
  State_Psi_q_GFL_15_c1e2a : Inport  Port=5
  Constant_Kqi_8b505 : Constant  Value=Kqi
  Constant_Tqi_0ac83 : Constant  Value=Tqi
  Constant_Vbase_3b5e8 : Constant  Value=Vbase
  Divide_6fe92 : Product  Inputs=*/
  MathFunc_cos_3e908 : Trigonometry  Operator=cos
  MathFunc_sin_87f81 : Trigonometry
  Product_42c6e : Product
  Product_6e8d4 : Product
  Product_7acd6 : Product
  Product_86d98 : Product
  Subtract_6f30b : Sum  Inputs=+-
  Subtract_7f230 : Sum  Inputs=+-
  Blockout_d_Psi_q_GFL_15_d79bb : Outport
  wires:
  State_theta_pll_GFL_15_42098/1 -> MathFunc_cos_3e908/1
  MathFunc_cos_3e908/1 -> Product_7acd6/2
  State_theta_pll_GFL_15_5b172/1 -> MathFunc_sin_87f81/1
  MathFunc_sin_87f81/1 -> Product_6e8d4/2
  Product_7acd6/1 -> Subtract_7f230/1
  Input_v_d_GFL_15_07bda/1 -> Product_7acd6/1
  Input_v_q_GFL_15_da40e/1 -> Product_6e8d4/1
  Constant_Kqi_8b505/1 -> Product_86d98/1
  Constant_Vbase_3b5e8/1 -> Product_86d98/2
  Product_6e8d4/1 -> Subtract_7f230/2
  Product_86d98/1 -> Product_42c6e/1
  Subtract_7f230/1 -> Product_42c6e/2
  Product_42c6e/1 -> Subtract_6f30b/1
  State_Psi_q_GFL_15_c1e2a/1 -> Subtract_6f30b/2
  Subtract_6f30b/1 -> Divide_6fe92/1
  Constant_Tqi_0ac83/1 -> Divide_6fe92/2
  Divide_6fe92/1 -> Blockout_d_Psi_q_GFL_15_d79bb/1
